simulink model "Fuel"  (R2018a)
settings: configuration reference "cs_ert" (kept outside this file)
settings Model: DataDictionary=Fuel.sldd  Creator=zhoutinglin  LastModifiedBy=zhoutinglin

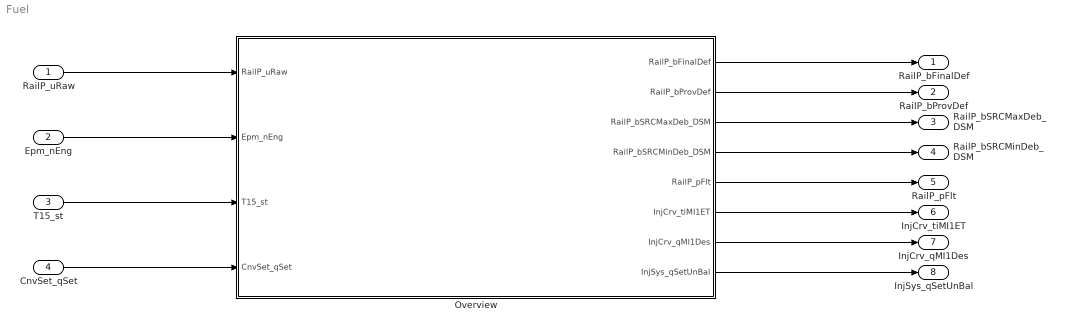
== system Fuel ==
  RailP_uRaw : Inport
  Epm_nEng : Inport  Port=2
  T15_st : Inport  Port=3
  CnvSet_qSet : Inport  Port=4
  Overview : Subsystem
  RailP_bFinalDef : Outport
  RailP_bProvDef : Outport  Port=2
  RailP_bSRCMaxDeb_DSM : Outport  Port=3
  RailP_bSRCMinDeb_DSM : Outport  Port=4
  RailP_pFlt : Outport  Port=5
  InjCrv_tiMI1ET : Outport  Port=6
  InjCrv_qMI1Des : Outport  Port=7
  InjSys_qSetUnBal : Outport  Port=8
  wires:
  RailP_uRaw/1 -> Overview/1(RailP_uRaw)
  Epm_nEng/1 -> Overview/2(Epm_nEng)
  T15_st/1 -> Overview/3(T15_st)
  CnvSet_qSet/1 -> Overview/4(CnvSet_qSet)
  Overview/1(RailP_bFinalDef) -> RailP_bFinalDef/1
  Overview/2(RailP_bProvDef) -> RailP_bProvDef/1
  Overview/3(RailP_bSRCMaxDeb_DSM) -> RailP_bSRCMaxDeb_DSM/1
  Overview/4(RailP_bSRCMinDeb_DSM) -> RailP_bSRCMinDeb_DSM/1
  Overview/5(RailP_pFlt) -> RailP_pFlt/1
  Overview/6(InjCrv_tiMI1ET) -> InjCrv_tiMI1ET/1
  Overview/7(InjCrv_qMI1Des) -> InjCrv_qMI1Des/1
  Overview/8(InjSys_qSetUnBal) -> InjSys_qSetUnBal/1

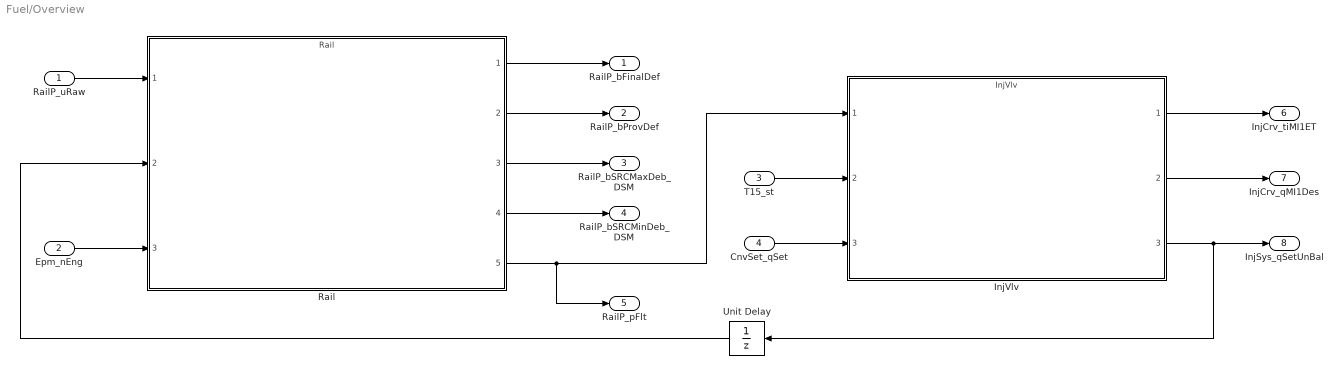
== system Fuel/Overview ==
  RailP_uRaw : Inport
  Epm_nEng : Inport  Port=2
  T15_st : Inport  Port=3
  CnvSet_qSet : Inport  Port=4
  InjVlv : ModelReference  ModelNameDialog=InjVlv  SimulationMode=Normal  ModelReferenceVersion=1.2
  Rail : ModelReference  ModelNameDialog=Rail  SimulationMode=Normal  ModelReferenceVersion=1.3
  Unit Delay : UnitDelay  SampleTime=-1
  RailP_bFinalDef : Outport
  RailP_bProvDef : Outport  Port=2
  RailP_bSRCMaxDeb_DSM : Outport  Port=3
  RailP_bSRCMinDeb_DSM : Outport  Port=4
  RailP_pFlt : Outport  Port=5
  InjCrv_tiMI1ET : Outport  Port=6
  InjCrv_qMI1Des : Outport  Port=7
  InjSys_qSetUnBal : Outport  Port=8
  wires:
  Rail/5 -> InjVlv/1, RailP_pFlt/1
  RailP_uRaw/1 -> Rail/1
  Epm_nEng/1 -> Rail/3
  Rail/1 -> RailP_bFinalDef/1
  Rail/2 -> RailP_bProvDef/1
  Rail/3 -> RailP_bSRCMaxDeb_DSM/1
  Rail/4 -> RailP_bSRCMinDeb_DSM/1
  T15_st/1 -> InjVlv/2
  CnvSet_qSet/1 -> InjVlv/3
  InjVlv/1 -> InjCrv_tiMI1ET/1
  InjVlv/2 -> InjCrv_qMI1Des/1
  InjVlv/3 -> Unit Delay/1, InjSys_qSetUnBal/1
  Unit Delay/1 -> Rail/2
